simulink model "gm_sampleModel1412_sub"  (R2023a)
settings: Solver=VariableStepAuto  StartTime=0.0  StopTime=10.0  RelTol=1e-3
libraries: simulink x1, hdlsllib x1
settings Model: Creator=user1  LastModifiedBy=user1
settings OptimizationCC: BlockReduction=off  ConditionallyExecuteInputs=off
settings DebuggingCC: InheritedTsInSrcMsg=none

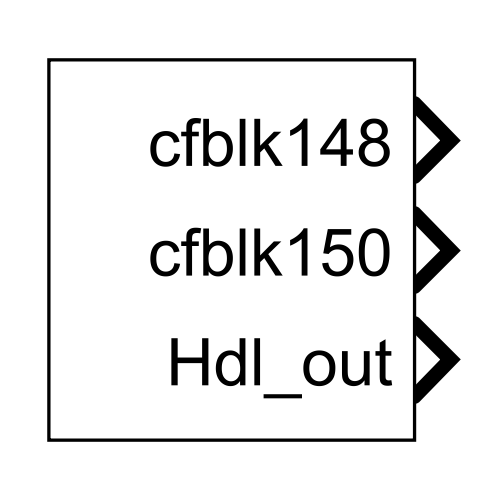
[thumbnail: Simulink's stored preview of the top-level diagram]
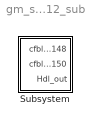
== system gm_sampleModel1412_sub ==
  Subsystem : Subsystem

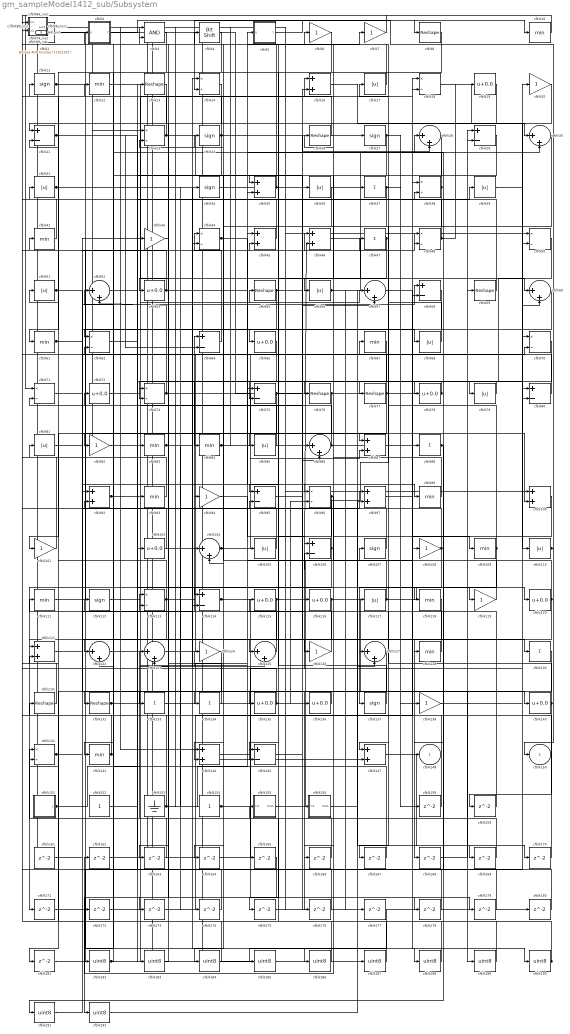
== system gm_sampleModel1412_sub/Subsystem ==
  cfblk1 : simulink/Logic and Bit Operations/Bitwise Operator  logicop=AND  UseBitMask=on  BitMask=bin2dec('11011001')  BitMaskRealWorld=Stored Integer
      settings: LibrarySourceBlock=|
      | hdlsllib/Logic and Bit
      | Operations/Bitwise
      | Operator
  cfblk{10,12,41,61,67,83..84,93,98,109,111,118,128,142} (14 alike) : MinMax  OutDataTypeStr=uint8
  cfblk{16,35,45..46,87,92,97,100,121,144,147} (11 alike) : Sum  OutDataTypeStr=uint8
  cfblk{6..7,20,43,82,94,101,108,119,124,126,138} (12 alike) : Gain  OutDataTypeStr=uint8
  cfblk102_inst : Subsystem
  cfblk{19,53,65,72,78,103,115..116,120,135..136,140} (12 alike) : Bias  Bias=0.0  SaturateOnIntegerOverflow=off
  cfblk{28,30,52,57,60,86,104,122..123,125,127} (11 alike) : Sum  Inputs=|++  OutDataTypeStr=uint8
  cfblk{17,31,36,39,51,56,68,79,81,85,105,110,117} (13 alike) : Abs  OutDataTypeStr=uint8  SaturateOnIntegerOverflow=off
  cfblk{21,29,58,64,75,80,95,106,114,145} (10 alike) : Sum  Inputs=+-  OutDataTypeStr=uint8
  cfblk{11,24,27,34,107,112,137} (7 alike) : Signum
  cfblk{14,18,23,38,44,48,50,62,70..71,73,96,113,141} (14 alike) : Product  Inputs=*/  OutDataTypeStr=uint8  RndMeth=Zero  SaturateOnIntegerOverflow=on
  cfblk{8,13,26,55,59,76..77,131..132} (9 alike) : Reshape
  cfblk{37,47,88,130,133..134} (6 alike) : Sum  Inputs=+  OutDataTypeStr=uint8
  cfblk139_inst : Subsystem
  cfblk151 : Subsystem  mask(Counter Free-Running){NumBits=double(16), tsamp=double(-1)}
      mask prompts: NumBits "Simulink:masks:NumberOfBits_MP"; tsamp "Simulink:masks:SampleTime_MP"
      mask help: Simulink:masks:CounterFreeRunning_MD
  cfblk152 : Constant  OutDataTypeStr=uint8  SampleTime=-1
  cfblk153 : Ground
  cfblk154 : Constant  OutDataTypeStr=uint8  SampleTime=-1
  cfblk155 : Subsystem
  cfblk156 : Subsystem
  cfblk{158..159,161..181} (23 alike) : Delay  SampleTime=1
  cfblk15_inst : Subsystem
  cfblk{182..192} (11 alike) : DataTypeConversion  OutDataTypeStr=uint8  SaturateOnIntegerOverflow=off  RndMeth=Floor
  cfblk2 : Subsystem  mask(Detect Fall Nonpositive){vinit=double(0), InputProcessing=Elements as channels (sample based), OutDataTypeStr=uint8}
      mask prompts: vinit "Simulink:masks:InitialCondition_MP"; InputProcessing "Simulink:masks:InputProcessing_MP"; OutDataTypeStr "Simulink:masks:OutputDataType_MP"
      mask help: Simulink:masks:DetectFallNonpositive_MD
      mask init:
      | InputProcessing = 'Elements as channels (sample based)';
      | OutDataTypeStr = 'uint8';
      | vinit = double(0);
      mask TypeOptions InputProcessing: Simulink:masks:ColumnsAsChannelsFrameBased | Simulink:masks:ElementsAsChannelsSampleBased
      mask TypeOptions OutDataTypeStr: Simulink:masks:uint8 | Simulink:masks:boolean
      mask Display: fprintf('U <= 0\n&  NOT\nU/z <= 0')
  cfblk25_inst : Subsystem
  cfblk3 : Logic  AllPortsSameDT=off  OutDataTypeStr=boolean
  cfblk32_inst : Subsystem
  cfblk33_inst : Subsystem
  cfblk4 : hdlsllib/Logic and Bit Operations/Bit Shift  mode=Shift Left Logical  N=0
  cfblk40_inst : Subsystem
  cfblk42_inst : Subsystem
  cfblk49_inst : Subsystem
  cfblk5 : Subsystem  mask(Detect Fall Nonpositive){vinit=double(0), InputProcessing=Elements as channels (sample based), OutDataTypeStr=uint8}
      mask prompts: vinit "Simulink:masks:InitialCondition_MP"; InputProcessing "Simulink:masks:InputProcessing_MP"; OutDataTypeStr "Simulink:masks:OutputDataType_MP"
      mask help: Simulink:masks:DetectFallNonpositive_MD
      mask init:
      | InputProcessing = 'Elements as channels (sample based)';
      | OutDataTypeStr = 'uint8';
      | vinit = double(0);
      mask TypeOptions InputProcessing: Simulink:masks:ColumnsAsChannelsFrameBased | Simulink:masks:ElementsAsChannelsSampleBased
      mask TypeOptions OutDataTypeStr: Simulink:masks:uint8 | Simulink:masks:boolean
      mask Display: fprintf('U <= 0\n&  NOT\nU/z <= 0')
  cfblk63_inst : Subsystem
  cfblk66_inst : Subsystem
  cfblk74_inst : Subsystem
  cfblk89_inst : Subsystem
  cfblk99_inst : Subsystem
  cfblk9_inst : Subsystem
  cfblk148 : Outport  OutDataTypeStr=uint8  SampleTime=1  VectorParamsAs1DForOutWhenUnconnected=off
  cfblk150 : Outport  Port=2  OutDataTypeStr=uint8  SampleTime=1  VectorParamsAs1DForOutWhenUnconnected=off
  Hdl_out : Outport  Port=3  OutDataTypeStr=uint8  SampleTime=1
  wires:
  cfblk1/1 -> cfblk186/1
  cfblk10/1 -> cfblk71/1
  cfblk100/1 -> cfblk162/1
  cfblk101/1 -> cfblk33_inst/2(in2)
  cfblk102_inst/1(out1) -> cfblk99_inst/2(in2)
  cfblk103/1 -> cfblk21/2
  cfblk104/1 -> cfblk87/2, cfblk67/1
  cfblk105/1 -> cfblk63_inst/1(in1)
  cfblk106/1 -> cfblk6/1, cfblk171/1
  cfblk107/1 -> cfblk9_inst/1(in1)
  cfblk108/1 -> cfblk64/1, cfblk137/1
  cfblk109/1 -> cfblk191/1, cfblk17/1
  cfblk11/1 -> cfblk68/1, cfblk130/1
  cfblk110/1 -> cfblk14/2, cfblk150/1
  cfblk111/1 -> cfblk46/1
  cfblk112/1 -> cfblk16/1
  cfblk113/1 -> cfblk95/2, cfblk121/1, cfblk11/1
  cfblk114/1 -> cfblk179/1, cfblk178/1
  cfblk115/1 -> cfblk46/2, cfblk122/1
  cfblk116/1 -> cfblk189/1, cfblk125/1
  cfblk117/1 -> cfblk26/1, cfblk119/1
  cfblk118/1 -> cfblk168/1
  cfblk119/1 -> cfblk32_inst/1(in1)
  cfblk12/1 -> cfblk60/1
  cfblk120/1 -> cfblk23/2, cfblk175/1, cfblk142/1
  cfblk121/1 -> cfblk58/1
  cfblk122/1 -> cfblk55/1
  cfblk123/1 -> cfblk45/1
  cfblk124/1 -> cfblk181/1
  cfblk125/1 -> cfblk112/1
  cfblk126/1 -> cfblk94/1
  cfblk127/1 -> cfblk176/1
  cfblk128/1 -> cfblk111/1
  cfblk13/1 -> cfblk132/1
  cfblk130/1 -> cfblk147/1
  cfblk131/1 -> cfblk74_inst/1(in1)
  cfblk132/1 -> cfblk125/2, cfblk48/1, cfblk124/1
  cfblk133/1 -> cfblk107/1
  cfblk134/1 -> cfblk92/2
  cfblk135/1 -> cfblk40_inst/1(in1), cfblk96/2
  cfblk136/1 -> cfblk134/1
  cfblk137/1 -> cfblk32_inst/2(in2)
  cfblk138/1 -> cfblk20/1
  cfblk139_inst/1(out1) -> cfblk27/1
  cfblk14/1 -> cfblk21/1
  cfblk140/1 -> cfblk115/1, cfblk159/1
  cfblk141/1 -> cfblk70/2, cfblk113/1
  cfblk142/1 -> cfblk89_inst/2(in2), cfblk81/1, cfblk12/1
  cfblk144/1 -> cfblk70/1
  cfblk145/1 -> cfblk36/1
  cfblk147/1 -> cfblk169/1
  cfblk15_inst/1(out1) -> cfblk105/1, cfblk88/1
  cfblk151/1(y) -> cfblk31/1, cfblk103/1
  cfblk152/1 -> cfblk93/1
  cfblk153/1 -> cfblk35/2, cfblk34/1, cfblk131/1
  cfblk154/1 -> cfblk59/1, cfblk106/2
  cfblk155/1(Out1) -> cfblk38/1
  cfblk156/1(Out1) -> cfblk117/1
  cfblk158/1 -> cfblk92/1
  cfblk159/1 -> cfblk71/2
  cfblk16/1 -> cfblk30/1
  cfblk161/1 -> cfblk45/2
  cfblk162/1 -> cfblk14/1
  cfblk163/1 -> cfblk141/1
  cfblk164/1 -> cfblk18/2
  cfblk165/1 -> cfblk192/1
  cfblk166/1 -> cfblk123/1
  cfblk167/1 -> cfblk52/1
  cfblk168/1 -> cfblk29/2
  cfblk169/1 -> cfblk62/2
  cfblk17/1 -> cfblk42_inst/2(in2)
  cfblk170/1 -> cfblk122/2
  cfblk171/1 -> cfblk50/2
  cfblk172/1 -> cfblk104/1
  cfblk173/1 -> cfblk58/2
  cfblk174/1 -> cfblk139_inst/1(in1)
  cfblk175/1 -> cfblk57/2
  cfblk176/1 -> cfblk66_inst/1(in1)
  cfblk177/1 -> cfblk185/1
  cfblk178/1 -> cfblk113/2
  cfblk179/1 -> cfblk38/2
  cfblk18/1 -> cfblk80/1
  cfblk180/1 -> cfblk121/2
  cfblk181/1 -> cfblk13/1
  cfblk182/1 -> cfblk72/1, cfblk116/1
  cfblk183/1 -> cfblk3/1
  cfblk184/1 -> cfblk3/2
  cfblk185/1 -> cfblk1/1
  cfblk186/1 -> cfblk141/2
  cfblk187/1 -> cfblk49_inst/1(in1)
  cfblk188/1 -> cfblk25_inst/1(in1)
  cfblk189/1 -> cfblk25_inst/2(in2)
  cfblk19/1 -> cfblk53/1
  cfblk190/1 -> cfblk49_inst/2(in2), cfblk155/1(In1)
  cfblk191/1 -> cfblk97/1
  cfblk192/1 -> cfblk97/2
  cfblk2/1(Y) -> cfblk10/1
  cfblk20/1 -> cfblk135/1
  cfblk21/1 -> cfblk80/2, cfblk64/2, cfblk35/1
  cfblk23/1 -> cfblk9_inst/2(in2), cfblk86/2
  cfblk24/1 -> cfblk28/2, cfblk15_inst/2(in2), cfblk73/2
  cfblk25_inst/1(out1) -> cfblk187/1
  cfblk26/1 -> cfblk40_inst/2(in2)
  cfblk27/1 -> cfblk104/2, cfblk158/1
  cfblk28/1 -> cfblk56/1
  cfblk29/1 -> cfblk62/1
  cfblk3/1 -> cfblk182/1
  cfblk30/1 -> cfblk77/1
  cfblk31/1 -> cfblk188/1, cfblk127/1
  cfblk32_inst/1(out1) -> cfblk147/2, cfblk23/1
  cfblk33_inst/1(out1) -> cfblk50/1
  cfblk34/1 -> cfblk4/1
  cfblk35/1 -> cfblk89_inst/1(in1), cfblk139_inst/2(in2), cfblk128/1
  cfblk36/1 -> cfblk144/2
  cfblk37/1 -> cfblk95/1, cfblk138/1
  cfblk38/1 -> cfblk114/1, cfblk2/1(U)
  cfblk39/1 -> cfblk110/1
  cfblk4/1 -> cfblk61/1
  cfblk40_inst/1(out1) -> cfblk165/1
  cfblk41/1 -> cfblk15_inst/1(in1)
  cfblk42_inst/1(out1) -> cfblk180/1
  cfblk43/1 -> cfblk173/1
  cfblk44/1 -> cfblk76/1, cfblk98/1
  cfblk45/1 -> cfblk66_inst/2(in2)
  cfblk46/1 -> cfblk60/2
  cfblk47/1 -> cfblk85/1, cfblk145/2
  cfblk48/1 -> cfblk63_inst/2(in2), cfblk19/1
  cfblk49_inst/1(out1) -> cfblk144/1
  cfblk5/1(Y) -> cfblk8/1
  cfblk50/1 -> cfblk79/1
  cfblk51/1 -> cfblk43/1, cfblk126/1
  cfblk52/1 -> cfblk120/1
  cfblk53/1 -> cfblk99_inst/1(in1), cfblk7/1
  cfblk55/1 -> cfblk114/2, cfblk18/1
  cfblk56/1 -> cfblk29/1, cfblk127/2, cfblk177/1
  cfblk57/1 -> cfblk109/1
  cfblk58/1 -> cfblk123/2
  cfblk59/1 -> cfblk24/1
  cfblk6/1 -> cfblk172/1
  cfblk60/1 -> cfblk82/1
  cfblk61/1 -> cfblk65/1, cfblk96/1
  cfblk62/1 -> cfblk183/1
  cfblk63_inst/1(out1) -> cfblk156/1(In1)
  cfblk64/1 -> cfblk44/1
  cfblk65/1 -> cfblk184/1
  cfblk66_inst/1(out1) -> cfblk136/1
  cfblk67/1 -> cfblk84/1
  cfblk68/1 -> cfblk42_inst/1(in1)
  cfblk7/1 -> cfblk33_inst/1(in1)
  cfblk70/1 -> cfblk167/1
  cfblk71/1 -> cfblk140/1
  cfblk72/1 -> cfblk5/1(U)
  cfblk73/1 -> cfblk52/2, cfblk100/2
  cfblk74_inst/1(out1) -> cfblk37/1
  cfblk75/1 -> cfblk86/1, cfblk101/1
  cfblk76/1 -> cfblk164/1, cfblk163/1
  cfblk77/1 -> cfblk102_inst/2(in2), cfblk133/1
  cfblk78/1 -> cfblk73/1, Hdl_out/1
  cfblk79/1 -> cfblk78/1
  cfblk8/1 -> cfblk75/2
  cfblk80/1 -> cfblk41/1
  cfblk81/1 -> cfblk87/1
  cfblk82/1 -> cfblk16/2
  cfblk83/1 -> cfblk44/2, cfblk174/1
  cfblk84/1 -> cfblk57/1, cfblk30/2
  cfblk85/1 -> cfblk75/1
  cfblk86/1 -> cfblk51/1, cfblk170/1
  cfblk87/1 -> cfblk108/1
  cfblk88/1 -> cfblk28/1, cfblk148/1
  cfblk89_inst/1(out1) -> cfblk83/1
  cfblk9_inst/1(out1) -> cfblk161/1
  cfblk92/1 -> cfblk39/1, cfblk48/2, cfblk47/1
  cfblk93/1 -> cfblk102_inst/1(in1)
  cfblk94/1 -> cfblk106/1
  cfblk95/1 -> cfblk118/1
  cfblk96/1 -> cfblk145/1, cfblk166/1
  cfblk97/1 -> cfblk190/1
  cfblk98/1 -> cfblk74_inst/2(in2)
  cfblk99_inst/1(out1) -> cfblk100/1

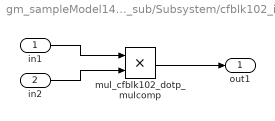
== system gm_sampleModel1412_sub/Subsystem/cfblk102_inst ==
  in1 : Inport  OutDataTypeStr=uint8  SampleTime=1
  in2 : Inport  Port=2  OutDataTypeStr=uint8  SampleTime=1
  mul_cfblk102_dotp_mulcomp : Product  Inputs=**  OutDataTypeStr=uint8  SampleTime=1
  out1 : Outport  OutDataTypeStr=uint8  SampleTime=1
  wires:
  in1/1 -> mul_cfblk102_dotp_mulcomp/1
  in2/1 -> mul_cfblk102_dotp_mulcomp/2
  mul_cfblk102_dotp_mulcomp/1 -> out1/1

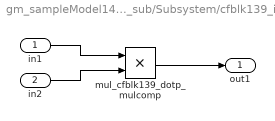
== system gm_sampleModel1412_sub/Subsystem/cfblk139_inst ==
  in1 : Inport  OutDataTypeStr=uint8  SampleTime=1
  in2 : Inport  Port=2  OutDataTypeStr=uint8  SampleTime=1
  mul_cfblk139_dotp_mulcomp : Product  Inputs=**  OutDataTypeStr=uint8  SampleTime=1
  out1 : Outport  OutDataTypeStr=uint8  SampleTime=1
  wires:
  in1/1 -> mul_cfblk139_dotp_mulcomp/1
  in2/1 -> mul_cfblk139_dotp_mulcomp/2
  mul_cfblk139_dotp_mulcomp/1 -> out1/1

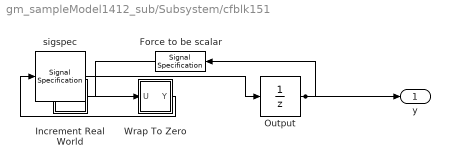
== system gm_sampleModel1412_sub/Subsystem/cfblk151 ==
  Force to be scalar : SignalSpecification  DisableCoverage=on  Dimensions=1
  Increment Real World : Subsystem  mask(Real World Value Increment){}
      mask help: Simulink:masks:RealWorldValueIncrement_MD
      mask Display: disp('V++')
  Output : UnitDelay  InitialCondition=0.0  SampleTime=tsamp  HasFrameUpgradeWarning=on
  Wrap To Zero : Subsystem  mask(Wrap To Zero){Threshold=double(65535)}
      mask prompts: Threshold "Simulink:masks:Threshold_MP"
      mask help: Simulink:masks:WrapToZero_MD
  sigspec : SignalSpecification  OutDataTypeStr=uint16  Dimensions=1
  y : Outport  SampleTime=1
  wires:
  Force to be scalar/1 -> Increment Real World/1(u)
  Increment Real World/1(y) -> Wrap To Zero/1(U)
  Output/1 -> Force to be scalar/1, y/1
  Wrap To Zero/1(Y) -> sigspec/1
  sigspec/1 -> Output/1

== system gm_sampleModel1412_sub/Subsystem/cfblk155 ==
  In1 : Inport  OutDataTypeStr=uint8  PortDimensions=1  SampleTime=1
  Out1 : Outport  SampleTime=1
  wires:
  In1/1 -> Out1/1

== system gm_sampleModel1412_sub/Subsystem/cfblk156 ==
  In1 : Inport  OutDataTypeStr=uint8  PortDimensions=1  SampleTime=1
  Out1 : Outport  SampleTime=1
  wires:
  In1/1 -> Out1/1

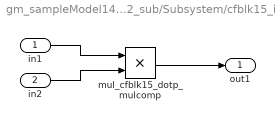
== system gm_sampleModel1412_sub/Subsystem/cfblk15_inst ==
  in1 : Inport  OutDataTypeStr=uint8  SampleTime=1
  in2 : Inport  Port=2  OutDataTypeStr=uint8  SampleTime=1
  mul_cfblk15_dotp_mulcomp : Product  Inputs=**  OutDataTypeStr=uint8  SampleTime=1
  out1 : Outport  OutDataTypeStr=uint8  SampleTime=1
  wires:
  in1/1 -> mul_cfblk15_dotp_mulcomp/1
  in2/1 -> mul_cfblk15_dotp_mulcomp/2
  mul_cfblk15_dotp_mulcomp/1 -> out1/1

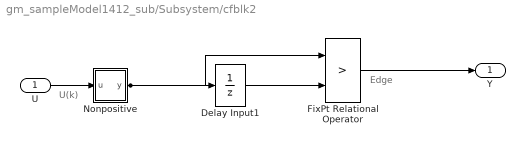
== system gm_sampleModel1412_sub/Subsystem/cfblk2 ==
  note: U(k)
  note: Edge
  U : Inport  OutDataTypeStr=uint8  SampleTime=1
  Delay Input1 : UnitDelay  Description=Store in Global RAM  DisableCoverage=on  InitialCondition=vinit  SampleTime=-1  HasFrameUpgradeWarning=on
  FixPt Relational Operator : RelationalOperator  Operator=>  OutDataTypeStr=fixdt(0, 8)  ZeroCross=off  InputSameDT=off
  Nonpositive : Subsystem  mask(Compare To Zero){relop=<=, OutDataTypeStr=boolean, ZeroCross=off}
      mask prompts: relop "Simulink:masks:Operator_MP"; OutDataTypeStr "Simulink:masks:OutputDataType_MP"; ZeroCross "Simulink:masks:EnableZerocrossingDetection_MP"
      mask help: Simulink:masks:CompareToZero_MD
      mask init:
      | OutDataTypeStr = 'boolean';
      | ZeroCross = 'off';
      | blkName = 'sampleModel1412_sub/Subsystem/cfblk2/Nonpositive';
      | relop = '<=';
      | setValue = 'boolean';
      mask TypeOptions relop: == | ~= | < | <= | >= | >
      mask TypeOptions OutDataTypeStr: Simulink:masks:uint8 | Simulink:masks:boolean
      mask Callback ZeroCross: sl('zeroCrossEnable', gcbh);
      mask Display: disp([relop,' 0'])
  Y : Outport  SampleTime=1
  wires:
  U/1 -> Nonpositive/1(u)
  Delay Input1/1 -> FixPt Relational Operator/2
  FixPt Relational Operator/1 -> Y/1
  Nonpositive/1(y) -> FixPt Relational Operator/1, Delay Input1/1

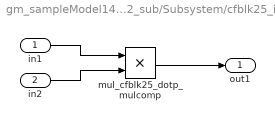
== system gm_sampleModel1412_sub/Subsystem/cfblk25_inst ==
  in1 : Inport  OutDataTypeStr=uint8  SampleTime=1
  in2 : Inport  Port=2  OutDataTypeStr=uint8  SampleTime=1
  mul_cfblk25_dotp_mulcomp : Product  Inputs=**  OutDataTypeStr=uint8  SampleTime=1
  out1 : Outport  OutDataTypeStr=uint8  SampleTime=1
  wires:
  in1/1 -> mul_cfblk25_dotp_mulcomp/1
  in2/1 -> mul_cfblk25_dotp_mulcomp/2
  mul_cfblk25_dotp_mulcomp/1 -> out1/1

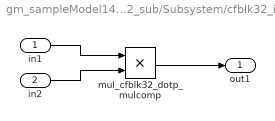
== system gm_sampleModel1412_sub/Subsystem/cfblk32_inst ==
  in1 : Inport  OutDataTypeStr=uint8  SampleTime=1
  in2 : Inport  Port=2  OutDataTypeStr=uint8  SampleTime=1
  mul_cfblk32_dotp_mulcomp : Product  Inputs=**  OutDataTypeStr=uint8  SampleTime=1
  out1 : Outport  OutDataTypeStr=uint8  SampleTime=1
  wires:
  in1/1 -> mul_cfblk32_dotp_mulcomp/1
  in2/1 -> mul_cfblk32_dotp_mulcomp/2
  mul_cfblk32_dotp_mulcomp/1 -> out1/1

== system gm_sampleModel1412_sub/Subsystem/cfblk33_inst ==
  in1 : Inport  OutDataTypeStr=uint8  SampleTime=1
  in2 : Inport  Port=2  OutDataTypeStr=uint8  SampleTime=1
  mul_cfblk33_dotp_mulcomp : Product  Inputs=**  OutDataTypeStr=uint8  SampleTime=1
  out1 : Outport  OutDataTypeStr=uint8  SampleTime=1
  wires:
  in1/1 -> mul_cfblk33_dotp_mulcomp/1
  in2/1 -> mul_cfblk33_dotp_mulcomp/2
  mul_cfblk33_dotp_mulcomp/1 -> out1/1

== system gm_sampleModel1412_sub/Subsystem/cfblk40_inst ==
  in1 : Inport  OutDataTypeStr=uint8  SampleTime=1
  in2 : Inport  Port=2  OutDataTypeStr=uint8  SampleTime=1
  mul_cfblk40_dotp_mulcomp : Product  Inputs=**  OutDataTypeStr=uint8  SampleTime=1
  out1 : Outport  OutDataTypeStr=uint8  SampleTime=1
  wires:
  in1/1 -> mul_cfblk40_dotp_mulcomp/1
  in2/1 -> mul_cfblk40_dotp_mulcomp/2
  mul_cfblk40_dotp_mulcomp/1 -> out1/1

== system gm_sampleModel1412_sub/Subsystem/cfblk42_inst ==
  in1 : Inport  OutDataTypeStr=uint8  SampleTime=1
  in2 : Inport  Port=2  OutDataTypeStr=uint8  SampleTime=1
  mul_cfblk42_dotp_mulcomp : Product  Inputs=**  OutDataTypeStr=uint8  SampleTime=1
  out1 : Outport  OutDataTypeStr=uint8  SampleTime=1
  wires:
  in1/1 -> mul_cfblk42_dotp_mulcomp/1
  in2/1 -> mul_cfblk42_dotp_mulcomp/2
  mul_cfblk42_dotp_mulcomp/1 -> out1/1

== system gm_sampleModel1412_sub/Subsystem/cfblk49_inst ==
  in1 : Inport  OutDataTypeStr=uint8  SampleTime=1
  in2 : Inport  Port=2  OutDataTypeStr=uint8  SampleTime=1
  mul_cfblk49_dotp_mulcomp : Product  Inputs=**  OutDataTypeStr=uint8  SampleTime=1
  out1 : Outport  OutDataTypeStr=uint8  SampleTime=1
  wires:
  in1/1 -> mul_cfblk49_dotp_mulcomp/1
  in2/1 -> mul_cfblk49_dotp_mulcomp/2
  mul_cfblk49_dotp_mulcomp/1 -> out1/1

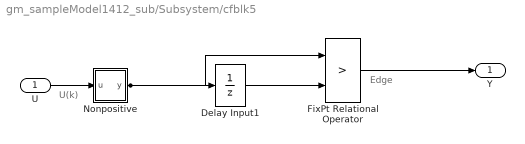
== system gm_sampleModel1412_sub/Subsystem/cfblk5 ==
  note: U(k)
  note: Edge
  U : Inport  OutDataTypeStr=uint8  SampleTime=1
  Delay Input1 : UnitDelay  Description=Store in Global RAM  DisableCoverage=on  InitialCondition=vinit  SampleTime=-1  HasFrameUpgradeWarning=on
  FixPt Relational Operator : RelationalOperator  Operator=>  OutDataTypeStr=fixdt(0, 8)  ZeroCross=off  InputSameDT=off
  Nonpositive : Subsystem  mask(Compare To Zero){relop=<=, OutDataTypeStr=boolean, ZeroCross=off}
      mask prompts: relop "Simulink:masks:Operator_MP"; OutDataTypeStr "Simulink:masks:OutputDataType_MP"; ZeroCross "Simulink:masks:EnableZerocrossingDetection_MP"
      mask help: Simulink:masks:CompareToZero_MD
      mask init:
      | OutDataTypeStr = 'boolean';
      | ZeroCross = 'off';
      | blkName = 'sampleModel1412_sub/Subsystem/cfblk5/Nonpositive';
      | relop = '<=';
      | setValue = 'boolean';
      mask TypeOptions relop: == | ~= | < | <= | >= | >
      mask TypeOptions OutDataTypeStr: Simulink:masks:uint8 | Simulink:masks:boolean
      mask Callback ZeroCross: sl('zeroCrossEnable', gcbh);
      mask Display: disp([relop,' 0'])
  Y : Outport  SampleTime=1
  wires:
  U/1 -> Nonpositive/1(u)
  Delay Input1/1 -> FixPt Relational Operator/2
  FixPt Relational Operator/1 -> Y/1
  Nonpositive/1(y) -> FixPt Relational Operator/1, Delay Input1/1

== system gm_sampleModel1412_sub/Subsystem/cfblk63_inst ==
  in1 : Inport  OutDataTypeStr=uint8  SampleTime=1
  in2 : Inport  Port=2  OutDataTypeStr=uint8  SampleTime=1
  mul_cfblk63_dotp_mulcomp : Product  Inputs=**  OutDataTypeStr=uint8  SampleTime=1
  out1 : Outport  OutDataTypeStr=uint8  SampleTime=1
  wires:
  in1/1 -> mul_cfblk63_dotp_mulcomp/1
  in2/1 -> mul_cfblk63_dotp_mulcomp/2
  mul_cfblk63_dotp_mulcomp/1 -> out1/1

== system gm_sampleModel1412_sub/Subsystem/cfblk66_inst ==
  in1 : Inport  OutDataTypeStr=uint8  SampleTime=1
  in2 : Inport  Port=2  OutDataTypeStr=uint8  SampleTime=1
  mul_cfblk66_dotp_mulcomp : Product  Inputs=**  OutDataTypeStr=uint8  SampleTime=1
  out1 : Outport  OutDataTypeStr=uint8  SampleTime=1
  wires:
  in1/1 -> mul_cfblk66_dotp_mulcomp/1
  in2/1 -> mul_cfblk66_dotp_mulcomp/2
  mul_cfblk66_dotp_mulcomp/1 -> out1/1

== system gm_sampleModel1412_sub/Subsystem/cfblk74_inst ==
  in1 : Inport  OutDataTypeStr=uint8  SampleTime=1
  in2 : Inport  Port=2  OutDataTypeStr=uint8  SampleTime=1
  mul_cfblk74_dotp_mulcomp : Product  Inputs=**  OutDataTypeStr=uint8  SampleTime=1
  out1 : Outport  OutDataTypeStr=uint8  SampleTime=1
  wires:
  in1/1 -> mul_cfblk74_dotp_mulcomp/1
  in2/1 -> mul_cfblk74_dotp_mulcomp/2
  mul_cfblk74_dotp_mulcomp/1 -> out1/1

== system gm_sampleModel1412_sub/Subsystem/cfblk89_inst ==
  in1 : Inport  OutDataTypeStr=uint8  SampleTime=1
  in2 : Inport  Port=2  OutDataTypeStr=uint8  SampleTime=1
  mul_cfblk89_dotp_mulcomp : Product  Inputs=**  OutDataTypeStr=uint8  SampleTime=1
  out1 : Outport  OutDataTypeStr=uint8  SampleTime=1
  wires:
  in1/1 -> mul_cfblk89_dotp_mulcomp/1
  in2/1 -> mul_cfblk89_dotp_mulcomp/2
  mul_cfblk89_dotp_mulcomp/1 -> out1/1

== system gm_sampleModel1412_sub/Subsystem/cfblk99_inst ==
  in1 : Inport  OutDataTypeStr=uint8  SampleTime=1
  in2 : Inport  Port=2  OutDataTypeStr=uint8  SampleTime=1
  mul_cfblk99_dotp_mulcomp : Product  Inputs=**  OutDataTypeStr=uint8  SampleTime=1
  out1 : Outport  OutDataTypeStr=uint8  SampleTime=1
  wires:
  in1/1 -> mul_cfblk99_dotp_mulcomp/1
  in2/1 -> mul_cfblk99_dotp_mulcomp/2
  mul_cfblk99_dotp_mulcomp/1 -> out1/1

== system gm_sampleModel1412_sub/Subsystem/cfblk9_inst ==
  in1 : Inport  OutDataTypeStr=uint8  SampleTime=1
  in2 : Inport  Port=2  OutDataTypeStr=uint8  SampleTime=1
  mul_cfblk9_dotp_mulcomp : Product  Inputs=**  OutDataTypeStr=uint8  SampleTime=1
  out1 : Outport  OutDataTypeStr=uint8  SampleTime=1
  wires:
  in1/1 -> mul_cfblk9_dotp_mulcomp/1
  in2/1 -> mul_cfblk9_dotp_mulcomp/2
  mul_cfblk9_dotp_mulcomp/1 -> out1/1

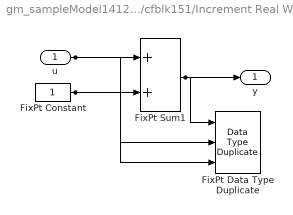
== system gm_sampleModel1412_sub/Subsystem/cfblk151/Increment Real World ==
  u : Inport  OutDataTypeStr=uint16  SampleTime=1
  FixPt Constant : Constant  DisableCoverage=on  OutDataTypeStr=Inherit: Inherit via back propagation  SampleTime=-1
  FixPt Data Type Duplicate : DataTypeDuplicate  DisableCoverage=on  NumInputPorts=3
  FixPt Sum1 : Sum  InputSameDT=on  OutDataTypeStr=Inherit: Inherit via back propagation  LockScale=on
  y : Outport  SampleTime=1
  wires:
  u/1 -> FixPt Sum1/1, FixPt Data Type Duplicate/2
  FixPt Constant/1 -> FixPt Sum1/2, FixPt Data Type Duplicate/3
  FixPt Sum1/1 -> FixPt Data Type Duplicate/1, y/1

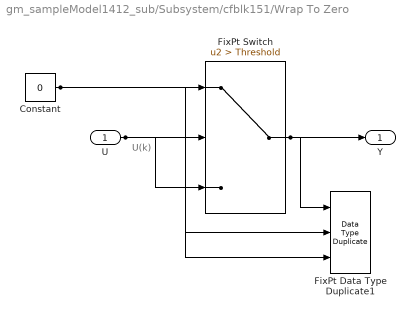
== system gm_sampleModel1412_sub/Subsystem/cfblk151/Wrap To Zero ==
  note: U(k)
  U : Inport  OutDataTypeStr=uint16  SampleTime=1
  Constant : Constant  DisableCoverage=on  Value=0  OutDataTypeStr=Inherit: Inherit via back propagation  SampleTime=-1
  FixPt Data Type Duplicate1 : DataTypeDuplicate  DisableCoverage=on  NumInputPorts=3
  FixPt Switch : Switch  Criteria=u2 > Threshold  Threshold=Threshold  OutDataTypeStr=Inherit: Inherit via back propagation  ZeroCross=off  SaturateOnIntegerOverflow=off  InputSameDT=off
  Y : Outport  SampleTime=1
  wires:
  U/1 -> FixPt Switch/3, FixPt Switch/2, FixPt Data Type Duplicate1/2
  Constant/1 -> FixPt Switch/1, FixPt Data Type Duplicate1/3
  FixPt Switch/1 -> FixPt Data Type Duplicate1/1, Y/1

== system gm_sampleModel1412_sub/Subsystem/cfblk2/Nonpositive ==
  u : Inport  OutDataTypeStr=uint8  SampleTime=1
  Compare : RelationalOperator  Operator=<=  OutDataTypeStr=boolean  ZeroCross=off
  Constant : Constant  DisableCoverage=on  Value=0  OutDataTypeStr=Inherit: Inherit via back propagation  SampleTime=-1  PreserveConstantTs=on
  y : Outport  SampleTime=1
  wires:
  u/1 -> Compare/1
  Compare/1 -> y/1
  Constant/1 -> Compare/2

== system gm_sampleModel1412_sub/Subsystem/cfblk5/Nonpositive ==
  u : Inport  OutDataTypeStr=uint8  SampleTime=1
  Compare : RelationalOperator  Operator=<=  OutDataTypeStr=boolean  ZeroCross=off
  Constant : Constant  DisableCoverage=on  Value=0  OutDataTypeStr=Inherit: Inherit via back propagation  SampleTime=-1  PreserveConstantTs=on
  y : Outport  SampleTime=1
  wires:
  u/1 -> Compare/1
  Compare/1 -> y/1
  Constant/1 -> Compare/2
